simulink model "SimplePendulum"  (R2022b)
settings: Solver=VariableStepAuto  StartTime=0.0  StopTime=10.0  MaxStep=1e-3  RelTol=1e-3
values from neighbouring files (symbols this model uses):
  g = 9.8    [SimplePendulum_main.m]
  L = lValues(i)    [SimplePendulum_main.m]
  q0 = 0.2    [SimplePendulum_main.m]
settings Model: Creator=Mo_7atem  LastModifiedBy=Mo_7atem

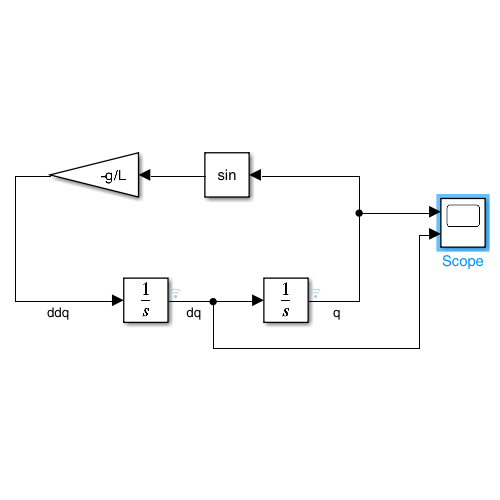
[thumbnail: Simulink's stored preview of the top-level diagram]
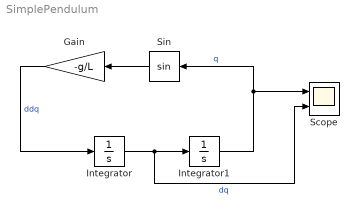
== system SimplePendulum ==
  Gain : Gain  Gain=-g/L
  Integrator : Integrator
  Integrator1 : Integrator  InitialCondition=q0
  Scope : Scope  NumInputPorts=2
  Sin : Trigonometry
  wires:
  Integrator/1 -> Scope/2, Integrator1/1  "dq"
  Gain/1 -> Integrator/1  "ddq"
  Integrator1/1 -> Sin/1, Scope/1  "q"
  Sin/1 -> Gain/1
